simulink model "PP2_JulioRibeiro"  (R2021b)
settings: Solver=VariableStepDiscrete  StartTime=0.0  StopTime=10.0  RelTol=1e-3
settings Model: Creator=julio-ribeiro  LastModifiedBy=julio-ribeiro

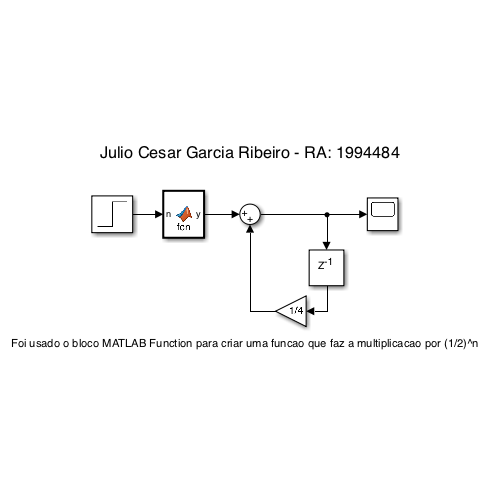
[thumbnail: Simulink's stored preview of the top-level diagram]
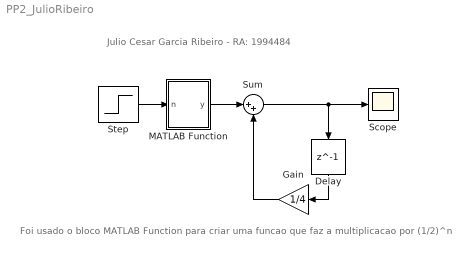
== system PP2_JulioRibeiro ==
  note: Foi usado o bloco MATLAB Function para criar uma funcao que faz a multiplicacao por (1/2)^n
  note: Julio Cesar Garcia Ribeiro - RA: 1994484
  Delay : Delay  DelayLength=1  InitialCondition=8
  Gain : Gain  Gain=1/4
  MATLAB Function : MATLAB Function  TreatAsAtomicUnit=on
  Scope : Scope
  Step : Step  SampleTime=0
  Sum : Sum  Inputs=|++
  wires:
  Delay/1 -> Gain/1
  Sum/1 -> Scope/1, Delay/1
  Gain/1 -> Sum/2
  MATLAB Function/1(y) -> Sum/1
  Step/1 -> MATLAB Function/1(n)

== matlab function PP2_JulioRibeiro/MATLAB Function ==
  data: n input; y output
function y = fcn(n)
    
y = (1/2)^n;
